simulink model "nivel0"  (R2020b)
settings: Solver=VariableStepAuto  StartTime=0.0  StopTime=10.0  RelTol=1e-3
settings Model: Creator=GoniR  LastModifiedBy=GoniR

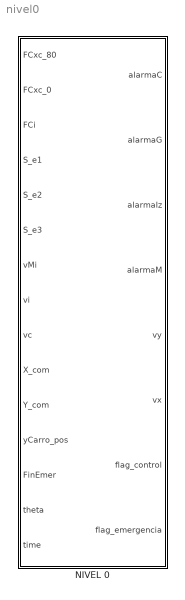
== system nivel0 ==
  NIVEL 0 : Stateflow chart  TreatAsAtomicUnit=on
      settings: PortSchema="{\"entries\":[{\"content\":{\"sides\":[{\"content\":{\"connectorIds\":[\"In1\",\"In2\",\"In3\",\"In4\",\"In5\",\"In6\",\"In7\",\"In8\",\"In9\",\"In11\",\"In12\",\"In13\",\"In14\",\"In15\",\"In10\"]},\"type\":\"ConnectorPlacement.EquallySpacedRectSide\",\"uuid\":\"257bd8b2-e50d-4f94-a780-554a728b2489\"},{\"content\":{\"connectorIds\":[\"Out1\",\"Out2\",\"Out3\",\"Out4\",\"Out5\",\"Out6\",\"Out7\",\"Out8\"],\"side\":\"RIGHT\"},\"type\":\"ConnectorPlacement.EquallySpacedRectSide\",\"uuid\":\"e3415bb4-ca91-4503-b89e-6184bd1dfb63\"},{\"content\":{\"connectorIds\":[],\"side\":\"TOP\"},\"type\":\"ConnectorPlacement.EquallySpacedRectSide\",\"uuid\":\"9a32744b-d02f-467d-83f2-39baa82bdd9b\"},{\"content\":{\"connectorIds\":[],\"side\":\"HIDDEN\"},\"type\":\"ConnectorPlacement.EquallySpacedRectSide\",\"uuid\":\"21a6614f-2711-4cba-b5d3-48b2ed3c7fdc\"}]},\"type\":\"ConnectorPlacement.EquallySpacedConnector\",\"uuid\":\"64bd3217-fe30-40b0-9b87-0656394712b6\"}],\"packageUris\":[\"http://schema.mathworks.com/mf0/Connector/R2020b\"],\"version\":\"1.0\"}"

== stateflow chart nivel0/NIVEL 0 ==
  state NORMAL
    state WATCHDOG [parallel]
      en:
      alarmaM=0;
      du:
      if(S_e1==0)
      alarmaM=1;
      end
      if(S_e2==0)
      alarmaM=1;
      end
      if(S_e3==0)
      alarmaM=1;
      end
      settings: executionOrder=2
    state CHEQUEO_ERROR [parallel]
      settings: executionOrder=1
      state Normal
        en:flag_emergencia=0;
        alarmaIz=0;
        alarmaC=0;
        alarmaG=0;
        flag_control=0;
      state ErrorIzaje
        en :
        alarmaIz=1;
      state ErrorCarro
        alarmaC=1;
      state ErrorGeneral
        alarmaG=1;
      (default) -> Normal
      Normal -> ErrorIzaje [order 1] : [FCi||vMi<vi]
      Normal -> ErrorCarro [order 2] : [FCxc_80 || FCxc_0 || vc>4]
      ErrorIzaje -> ErrorGeneral : [[FCxc_80 || FCxc_0 || vc>4]]
      ErrorCarro -> ErrorGeneral : [[FCi||vMi<vi]]
  state EMERGENCIA
    state ReduVeltransicion1
      en:
      flag_control=1;
      time_a=time;
      delta_t=0;
      vx=vc;
      vy=vi;
      du:
      delta_t=time-time_a;
      [vx,vy]=Calc_v1(delta_t,vx,vy)
      time_a=time;
      ex:
      vx = 0
      vy = 0
    state EstadoManual
      en :
      time_a=time;
      vx_a=0;
      vy_a=0;
      delta_t=0;
      flag_emergencia=1;
      du :
      delta_t=time-time_a;
      [vx,vy]=Calc_v(delta_t,vx_a,vy_a,X_com,Y_com);
      time_a=time;
      vx_a=vx;
      vy_a=vy;
    state Apagar_alarm
      en:
      alarmaIz=0;
      alarmaC=0;
      alarmaG=0;
      alarmaM=0
    (default) -> ReduVeltransicion1
    ReduVeltransicion1 -> EstadoManual : [abs(vx)<0.1 && abs(vy)<0.01 && theta<0.05]
    EstadoManual -> Apagar_alarm : [FinEmer]
  (default) -> NORMAL
  NORMAL -> EMERGENCIA : [alarmaM||alarmaG||alarmaC||alarmaIz]
  EMERGENCIA -> NORMAL : [alarmaM==0&&alarmaG==0&&alarmaC==0&&alarmaIz==0]
  data: delta_t2 function_input double; vx_a2 function_input double; vy_a2 function_input double; vx2 function_output; vy2 function_output; delta_t1 function_input double; vx_a1 function_input double; vy_a1 function_input double; vx1 function_output; vy1 function_output; X_com1 function_input; Y_com1 function_input; FCxc_80 input; FCxc_0 input; FCi input; S_e1 input; S_e2 input; S_e3 input; vMi input; vi input; vc input; time input; X_com input; Y_com input; yCarro_pos input; alarmaC output; alarmaG output; alarmaIz output; alarmaM output; time_a local; vx_a local; vy_a local; delta_t local; vy output; vx output; FinEmer input; flag_control output; flag_emergencia output; theta input
  function [vx2,vy2]=Calc_v1(delta_t2,vx_a2,vy_a2):
    | function [vx2,vy2]=Calc_v1(delta_t2,vx_a2,vy_a2)
    | if (vx_a2 < 0 )
    |     vx2=0.2*(delta_t2)+vx_a2;
    | else
    |     vx2=-0.2*(delta_t2)+vx_a2;
    | end
    | if (vy_a2 < 0)
    |     vy2=0.2*(delta_t2)+vy_a2
    | else
    |     vy2=-0.2*(delta_t2)+vy_a2
    | end
    | end
  function [vx1,vy1]=Calc_v(delta_t1,vx_a1,vy_a1,X_com1,Y_com1):
    | function [vx1,vy1]=Calc_v(delta_t1,vx_a1,vy_a1,X_com1,Y_com1)
    | if (X_com1 == 29 && vx_a1<4)
    |     vx1=0.8*(delta_t1)+vx_a1;
    | elseif (X_com1 == 28 && vx_a1 > -4 )
    |     vx1=-0.8*(delta_t1)+vx_a1;
    | else
    |     vx1=vx_a1;
    | end
    | if (Y_com1 == 31 && vy_a1<1.5)
    |     vy1=0.8*(delta_t1)+vy_a1
    | elseif (Y_com1==30 && vy_a1>-1.5)
    |     vy1=-0.8*(delta_t1)+vy_a1
    | else
    |     vy1=vy_a1
    | end
    | 
    | end
